simulink model "Sistem"  (R2019b)
settings: Solver=VariableStepAuto  StartTime=0.0  StopTime=50  RelTol=1e-3
values from neighbouring files (symbols this model uses):
  k = 0.035    [part1.m]
  k11 = k2^2+4*(k-k3)*k1    (= 0.0933546)    [part1.m]
  k12 = 8*(k-k3)    (= 0.2848)    [part1.m]
  k13 = 2*(k-k3)    (= 0.0712)    [part1.m]
  k2 = -0.015    [part1.m]
  keta = 8e-5    (= 8e-05)    [part1.m]
settings Model: Creator=ovi  LastModifiedBy=ovi

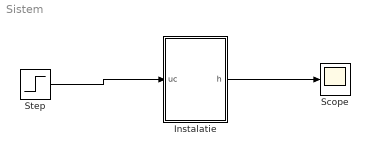
== system Sistem ==
  "Instalatie " : Subsystem
  Scope : Scope
  Step : Step  After=5  SampleTime=0
  wires:
  Step/1 -> "Instalatie "/1(uc)
  "Instalatie "/1(h) -> Scope/1

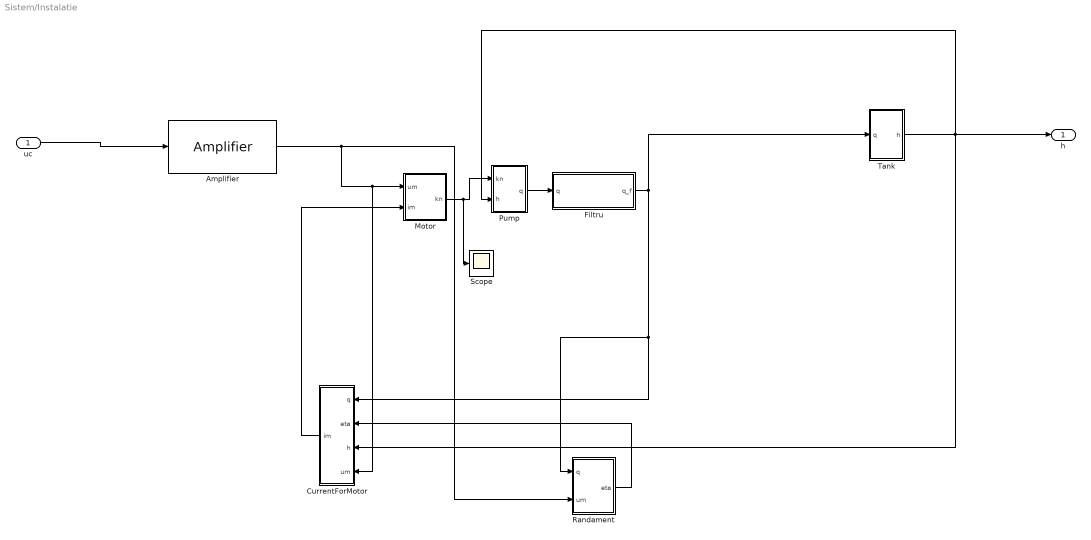
== system Sistem/Instalatie  ==
  uc : Inport
  Amplifier : MATLABFcn  MATLABFcn=Amplifier
  CurrentForMotor : Subsystem
  "Filtru " : Subsystem
  "Motor " : Subsystem
  Pump : Subsystem
  Randament : Subsystem
  Scope : Scope
  "Tank " : Subsystem
  h : Outport
  wires:
  "Tank "/1(h) -> Pump/2(h), h/1, CurrentForMotor/3("h ")
  "Filtru "/1(q_f) -> Randament/1(q), CurrentForMotor/1(q), "Tank "/1(q)
  Pump/1(q) -> "Filtru "/1(q)
  "Motor "/1(kn) -> Scope/1, Pump/1(kn)
  CurrentForMotor/1(im) -> "Motor "/2(im)
  uc/1 -> Amplifier/1
  Randament/1(eta) -> CurrentForMotor/2(eta)
  Amplifier/1 -> CurrentForMotor/4(um), "Motor "/1(um), Randament/2("um ")

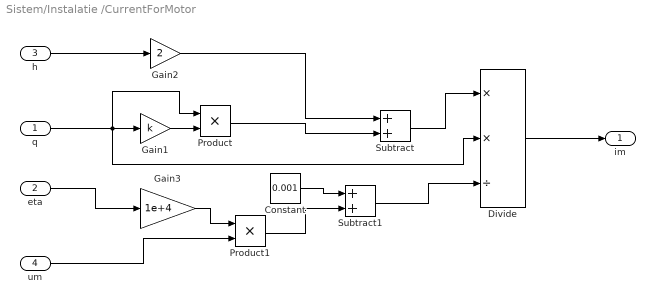
== system Sistem/Instalatie /CurrentForMotor ==
  q : Inport
  eta : Inport  Port=2
  "h " : Inport  Port=3
  um : Inport  Port=4
  Constant : Constant  Value=0.001
  Divide : Product  Inputs=**/
  Gain1 : Gain  Gain=k
  Gain2 : Gain  Gain=2
  Gain3 : Gain  Gain=1e+4
  Product : Product
  Product1 : Product
  Subtract : Sum
  Subtract1 : Sum
  im : Outport
  wires:
  eta/1 -> Gain3/1
  Gain3/1 -> Product1/1
  "h "/1 -> Gain2/1
  Gain2/1 -> Subtract/1
  Subtract/1 -> Divide/1
  Constant/1 -> Subtract1/1
  Product1/1 -> Subtract1/2
  Gain1/1 -> Product/2
  um/1 -> Product1/2
  Product/1 -> Subtract/2
  Subtract1/1 -> Divide/3
  q/1 -> Divide/2, Product/1, Gain1/1
  Divide/1 -> im/1

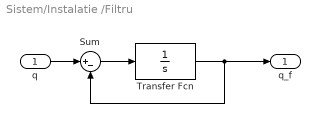
== system Sistem/Instalatie /Filtru  ==
  q : Inport
  Sum : Sum  Inputs=|+-
  Transfer Fcn : TransferFcn  Denominator=[1 0]
  q_f : Outport
  wires:
  q/1 -> Sum/1
  Sum/1 -> Transfer Fcn/1
  Transfer Fcn/1 -> Sum/2, q_f/1

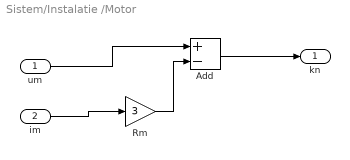
== system Sistem/Instalatie /Motor  ==
  um : Inport
  im : Inport  Port=2
  Add : Sum  Inputs=+-
  Rm : Gain  Gain=3
  kn : Outport
  wires:
  Rm/1 -> Add/2
  im/1 -> Rm/1
  um/1 -> Add/1
  Add/1 -> kn/1

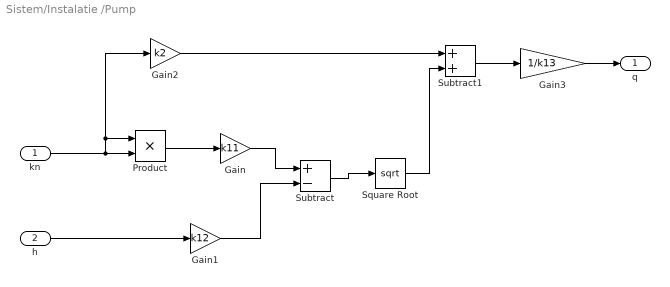
== system Sistem/Instalatie /Pump ==
  kn : Inport
  h : Inport  Port=2
  Gain : Gain  Gain=k11
  Gain1 : Gain  Gain=k12
  Gain2 : Gain  Gain=k2
  Gain3 : Gain  Gain=1/k13
  Product : Product
  Square Root : Sqrt  SaturateOnIntegerOverflow=on
  Subtract : Sum  Inputs=+-
  Subtract1 : Sum
  q : Outport
  wires:
  Gain/1 -> Subtract/1
  Gain2/1 -> Subtract1/1
  Subtract1/1 -> Gain3/1
  h/1 -> Gain1/1
  Product/1 -> Gain/1
  Subtract/1 -> Square Root/1
  Square Root/1 -> Subtract1/2
  kn/1 -> Gain2/1, Product/1, Product/2
  Gain1/1 -> Subtract/2
  Gain3/1 -> q/1

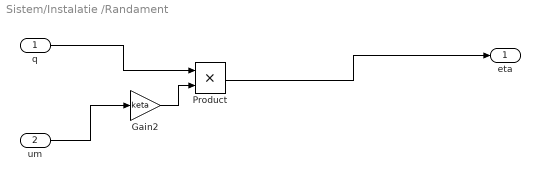
== system Sistem/Instalatie /Randament ==
  q : Inport
  "um " : Inport  Port=2
  Gain2 : Gain  Gain=keta
  Product : Product
  eta : Outport
  wires:
  q/1 -> Product/1
  Gain2/1 -> Product/2
  "um "/1 -> Gain2/1
  Product/1 -> eta/1

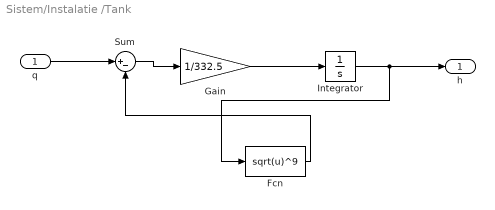
== system Sistem/Instalatie /Tank  ==
  q : Inport
  Fcn : Fcn  Expr=sqrt(u)^9
  Gain : Gain  Gain=1/332.5
  Integrator : Integrator
  Sum : Sum  Inputs=|+-
  h : Outport
  wires:
  Fcn/1 -> Sum/2
  q/1 -> Sum/1
  Integrator/1 -> h/1, Fcn/1
  Gain/1 -> Integrator/1
  Sum/1 -> Gain/1
